simulink model "HydroEye_6DOF_HITL"  (R2024b)
settings: Solver=VariableStepAuto  StartTime=0.0  StopTime=1200  RelTol=1e-3
undefined symbols (not defined in the file): alpha_vec_Cn0, b, b_ref, beta_vec_Cn0, c, CD_flaps, CDo_CD_elev, cg, CL_flaps, Clbeta, Clda, CLo_CL_elev, Clo_Cl_rudder, Clp, Clr, Cm0, Cm_flaps, Cmda, Cmde, Cmo_Cm_elev, Cmq, Cn0, Cnda, Cno_Cn_rudder, Cnp, Cnr, contact, control, cp, CX0, CXda, CXde, CYbeta, CYda, Cyo_Cy_rudder, CZ0, CZda, CZde, d_ref, Earth, F, fractalcoef, Light, m_to_mm, mass, MIL, ms_to_cms, Payload, ref_height, ref_lat, ref_lon, SampleTime, uT_to_gauss, WGS84
libraries: uavmavlinklib x7, simulink_extras x4, aerolibwind2 x3, aerolibatmos2 x2, aerolibasang x2, px4MAVLinkBridgelib x2, shared6dof x1, aerolibadyn x1, simulink x1, aerolibtransform2 x1, sensorgpslib x1, robotcorelib x1
(part 2 of 2)

== system HydroEye_6DOF_HITL/HydroEye Dynamics/Aerodynamics/Aerodynamic Coefficients/Actuator Increments ==
  Alpha : Inport  Unit=deg
  "Actuator Deflections " : Inport  Port=2  Unit=deg
  (0 to inf) Constants Held fixed for alpha<0 : Saturate  UpperLimit=inf  LowerLimit=0
  Ailerons : Subsystem
  AlphaLookup : PreLookup  BreakpointsData=alpha_vec_0  BeginIndexSearchUsingPreviousIndexResult=on  ExtrapMethod=Linear
  AlphaLookup0 : PreLookup  BreakpointsData=alpha_vec_0  BeginIndexSearchUsingPreviousIndexResult=on  ExtrapMethod=Linear
  Bus Creator : BusCreator  Inputs=2
  Bus Creator1 : BusCreator  Inputs=2
  Ruddervators : Subsystem
  Sum : Sum  InputSameDT=on  SaturateOnIntegerOverflow=on  OutDataTypeStr=Inherit: Same as first input
  cl : Outport  InitialOutput=0  VectorParamsAs1DForOutWhenUnconnected=off
  wires:
  Bus Creator/1 -> Ailerons/1(Alpha)
  (0 to inf) Constants Held fixed for alpha<0/1 -> AlphaLookup0/1
  "Actuator Deflections "/1 -> Ailerons/2(Actuators), Ruddervators/2(Actuators)
  Alpha/1 -> (0 to inf) Constants Held fixed for alpha<0/1, AlphaLookup/1
  Ailerons/1(delCoeff) -> Sum/1
  Ruddervators/1(delCoeff) -> Sum/2
  Sum/1 -> cl/1
  Bus Creator1/1 -> Ruddervators/1(Alpha)
  AlphaLookup0/1 -> Bus Creator/1  "k"
  AlphaLookup0/2 -> Bus Creator/2  "f"
  AlphaLookup/1 -> Bus Creator1/1  "k"
  AlphaLookup/2 -> Bus Creator1/2  "f"

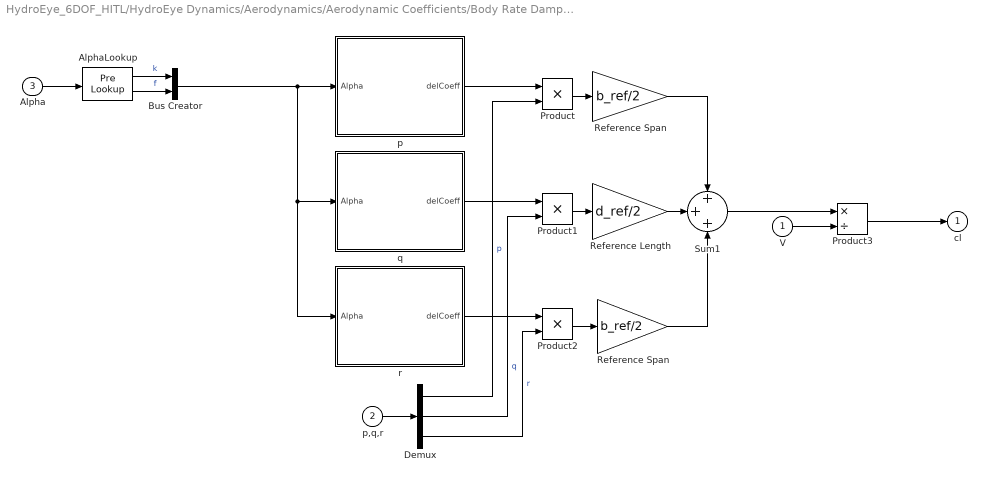
== system HydroEye_6DOF_HITL/HydroEye Dynamics/Aerodynamics/Aerodynamic Coefficients/Body Rate Damping ==
  V : Inport  Unit=m/s
  p,q,r : Inport  Port=2  Unit=rad/second
  Alpha : Inport  Port=3  Unit=deg
  AlphaLookup : PreLookup  BreakpointsData=alpha_vec_damping  BeginIndexSearchUsingPreviousIndexResult=on  ExtrapMethod=Linear
  Bus Creator : BusCreator  Inputs=2
  Demux : Demux  Outputs=3
      settings: DisplayOption=none
  Product : Product  InputSameDT=on  SaturateOnIntegerOverflow=on  OutDataTypeStr=Inherit: Same as first input
  Product1 : Product  InputSameDT=on  SaturateOnIntegerOverflow=on  OutDataTypeStr=Inherit: Same as first input
  Product2 : Product  InputSameDT=on  SaturateOnIntegerOverflow=on  OutDataTypeStr=Inherit: Same as first input
  Product3 : Product  Inputs=*/  InputSameDT=on  SaturateOnIntegerOverflow=on  OutDataTypeStr=Inherit: Same as first input
  Reference Length : Gain  Gain=d_ref/2  SaturateOnIntegerOverflow=on  OutDataTypeStr=Inherit: Same as input  ParamDataTypeStr=Inherit: Same as input
  Reference Span : Gain  Gain=b_ref/2  SaturateOnIntegerOverflow=on  OutDataTypeStr=Inherit: Same as input  ParamDataTypeStr=Inherit: Same as input
  "Reference Span " : Gain  Gain=b_ref/2  SaturateOnIntegerOverflow=on  OutDataTypeStr=Inherit: Same as input  ParamDataTypeStr=Inherit: Same as input
  Sum1 : Sum  Inputs=+++  InputSameDT=on  SaturateOnIntegerOverflow=on  OutDataTypeStr=Inherit: Same as first input
  p : Subsystem
  q : Subsystem
  r : Subsystem
  cl : Outport  InitialOutput=0  VectorParamsAs1DForOutWhenUnconnected=off
  wires:
  Alpha/1 -> AlphaLookup/1
  p/1(delCoeff) -> Product/1
  q/1(delCoeff) -> Product1/1
  p,q,r/1 -> Demux/1
  Demux/1 -> Product/2  "p"
  Demux/2 -> Product1/2  "q"
  Demux/3 -> Product2/2  "r"
  Sum1/1 -> Product3/1
  V/1 -> Product3/2
  Product3/1 -> cl/1
  Product1/1 -> Reference Length/1
  Product2/1 -> "Reference Span "/1
  Product/1 -> Reference Span/1
  r/1(delCoeff) -> Product2/1
  Bus Creator/1 -> r/1(Alpha), q/1(Alpha), p/1(Alpha)
  Reference Length/1 -> Sum1/2
  Reference Span/1 -> Sum1/1
  "Reference Span "/1 -> Sum1/3
  AlphaLookup/1 -> Bus Creator/1  "k"
  AlphaLookup/2 -> Bus Creator/2  "f"

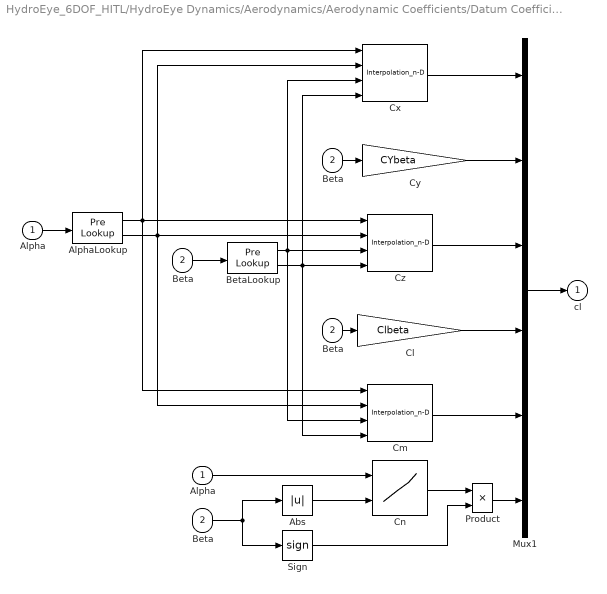
== system HydroEye_6DOF_HITL/HydroEye Dynamics/Aerodynamics/Aerodynamic Coefficients/Datum Coefficients ==
  Alpha : Inport  Unit=deg
  Beta : Inport  Port=2  Unit=deg
  " Cn" : Lookup_n-D  BreakpointsForDimension1=alpha_vec_Cn0  BreakpointsForDimension2=beta_vec_Cn0  Table=Cn0  InternalRulePriority=Speed  RndMeth=Simplest
      settings: InputPortMap=u0,u1
  " Beta" : InportShadow  Port=2  Unit=deg
  " Beta " : InportShadow  Port=2  Unit=deg
  Abs : Abs
  "Alpha " : InportShadow  Unit=deg
  AlphaLookup : PreLookup  BreakpointsData=alpha_vec_0  BeginIndexSearchUsingPreviousIndexResult=on  ExtrapMethod=Linear
  "Beta " : InportShadow  Port=2  Unit=deg
  BetaLookup : PreLookup  BreakpointsData=beta_vec_0  BeginIndexSearchUsingPreviousIndexResult=on  ExtrapMethod=Linear
  Cl : Gain  Gain=Clbeta  SaturateOnIntegerOverflow=on  OutDataTypeStr=Inherit: Same as input  ParamDataTypeStr=Inherit: Same as input
  Cm : Interpolation_n-D  Table=Cm0'  RemoveProtectionIndex=on
  Cx : Interpolation_n-D  Table=CX0'  RemoveProtectionIndex=on
  Cy : Gain  Gain=CYbeta  SaturateOnIntegerOverflow=on  OutDataTypeStr=Inherit: Same as input  ParamDataTypeStr=Inherit: Same as input
  Cz : Interpolation_n-D  Table=CZ0'  RemoveProtectionIndex=on
  Mux1 : Mux  Inputs=6
  Product : Product  InputSameDT=on  SaturateOnIntegerOverflow=on  OutDataTypeStr=Inherit: Same as first input
  Sign : Signum
  cl : Outport  InitialOutput=0  VectorParamsAs1DForOutWhenUnconnected=off
  wires:
  Sign/1 -> Product/2
  " Cn"/1 -> Product/1
  Product/1 -> Mux1/6
  Abs/1 -> " Cn"/2
  Mux1/1 -> cl/1
  Cx/1 -> Mux1/1
  Cz/1 -> Mux1/3
  Cm/1 -> Mux1/5
  Cy/1 -> Mux1/2
  Cl/1 -> Mux1/4
  Alpha/1 -> AlphaLookup/1
  Beta/1 -> BetaLookup/1
  AlphaLookup/1 -> Cz/1, Cm/1, Cx/1
  BetaLookup/1 -> Cz/3, Cx/3, Cm/3
  AlphaLookup/2 -> Cx/2, Cm/2, Cz/2
  "Beta "/1 -> Cy/1
  "Alpha "/1 -> " Cn"/1
  " Beta"/1 -> Abs/1, Sign/1
  " Beta "/1 -> Cl/1
  BetaLookup/2 -> Cz/4, Cx/4, Cm/4

== system HydroEye_6DOF_HITL/HydroEye Dynamics/Ground Model/Crash Detector/norm1 ==
  F : Inport
  Dot Product : DotProduct  OutDataTypeStr=Inherit: Inherit via internal rule
  Sqrt : Sqrt
  Out1 : Outport
  wires:
  Dot Product/1 -> Sqrt/1
  F/1 -> Dot Product/2, Dot Product/1
  Sqrt/1 -> Out1/1

== system HydroEye_6DOF_HITL/HydroEye Dynamics/Ground Model/Friction Force/Soft Coulomb Friction ==
  note: Pennestrì, E., Rossi, V., Salvini, P. et al. Review and comparison of dry friction force models. Nonlinear Dyn 83, 1785–1801 (2016). https://doi.org/10.1007/s11071-015-2485-3
  In1 : Inport
  Tanh : Trigonometry  Operator=tanh
  friction coefficient : Gain  Gain=contact.translation.friction
  vd : Gain  Gain=1/contact.translation.vd
  Out1 : Outport
  wires:
  In1/1 -> vd/1
  vd/1 -> Tanh/1
  Tanh/1 -> friction coefficient/1
  friction coefficient/1 -> Out1/1

== system HydroEye_6DOF_HITL/HydroEye Dynamics/Ground Model/Ground Moment Model/Soft Coulomb Friction ==
  note: Pennestrì, E., Rossi, V., Salvini, P. et al. Review and comparison of dry friction force models. Nonlinear Dyn 83, 1785–1801 (2016). https://doi.org/10.1007/s11071-015-2485-3
  In1 : Inport
  Tanh : Trigonometry  Operator=tanh
  friction coefficient : Gain  Gain=control.rotation.friction
  vd : Gain  Gain=1/control.rotation.vd
  Out1 : Outport
  wires:
  In1/1 -> vd/1
  vd/1 -> Tanh/1
  Tanh/1 -> friction coefficient/1
  friction coefficient/1 -> Out1/1

== system HydroEye_6DOF_HITL/HydroEye Dynamics/Aerodynamics/Aero Coeff/Damping Coeff/p & r ==
  <Angle Rate> : Inport
  <Vb> : Inport  Port=2
  Constant : Constant  Value=[Clp 0 Clr; Cnp 0 Cnr]
  Divide : Product  Inputs=*/
  Dot Product : DotProduct  OutDataTypeStr=Inherit: Inherit via internal rule
  Gain1 : Gain  Gain=b
  Gain2 : Gain  Gain=2
  Matrix Multiply : Product  Multiplication=Matrix(*)
  Radians to Degrees : simulink_extras/Transformations/Radians to Degrees
  Sqrt : Sqrt
  roll rate damping : Outport
  wires:
  Gain2/1 -> Divide/2
  Matrix Multiply/1 -> Gain1/1
  Gain1/1 -> Divide/1
  Divide/1 -> roll rate damping/1  "roll rate damping"
  Constant/1 -> Matrix Multiply/1
  <Vb>/1 -> Dot Product/1, Dot Product/2
  Dot Product/1 -> Sqrt/1
  Sqrt/1 -> Gain2/1
  <Angle Rate>/1 -> Radians to Degrees/1
  Radians to Degrees/1 -> Matrix Multiply/2

== system HydroEye_6DOF_HITL/HydroEye Dynamics/Aerodynamics/Aero Coeff/Damping Coeff/q ==
  <Angle Rate> : Inport
  <Vb> : Inport  Port=2
  Divide : Product  Inputs=*/
  Dot Product : DotProduct  OutDataTypeStr=Inherit: Inherit via internal rule
  Gain : Gain  Gain=Cmq
  Gain1 : Gain  Gain=c
  Gain2 : Gain  Gain=2
  Radians to Degrees : simulink_extras/Transformations/Radians to Degrees
  Selector : Selector  InputPortWidth=3  IndexOptions=Index vector (dialog)  Indices=2  OutputSizes=1
  pitch rate damping : Outport
  wires:
  Selector/1 -> Gain/1
  Gain2/1 -> Divide/2
  Gain/1 -> Gain1/1
  Gain1/1 -> Divide/1
  Divide/1 -> pitch rate damping/1  "pitch rate damping"
  <Vb>/1 -> Dot Product/1, Dot Product/2
  Dot Product/1 -> Gain2/1
  <Angle Rate>/1 -> Radians to Degrees/1
  Radians to Degrees/1 -> Selector/1

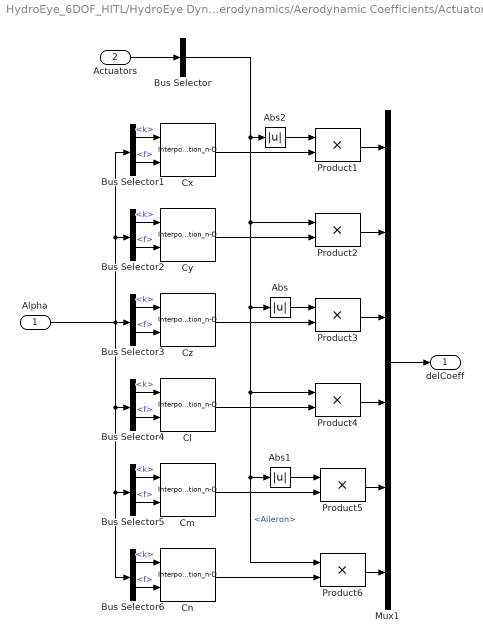
== system HydroEye_6DOF_HITL/HydroEye Dynamics/Aerodynamics/Aerodynamic Coefficients/Actuator Increments/Ailerons ==
  Alpha : Inport
  Actuators : Inport  Port=2
  Abs : Abs
  Abs1 : Abs
  Abs2 : Abs
  Bus Selector : BusSelector  OutputSignals=Aileron
  Bus Selector{1..6} (6 alike) : BusSelector  OutputSignals=k,f
  Cl : Interpolation_n-D  NumberOfTableDimensions=1  Table=Clda  RemoveProtectionIndex=on
      settings: InputPortMap=u0,u1
  Cm : Interpolation_n-D  NumberOfTableDimensions=1  Table=Cmda  RemoveProtectionIndex=on
      settings: InputPortMap=u0,u1
  Cn : Interpolation_n-D  NumberOfTableDimensions=1  Table=Cnda  RemoveProtectionIndex=on
      settings: InputPortMap=u0,u1
  Cx : Interpolation_n-D  NumberOfTableDimensions=1  Table=CXda  RemoveProtectionIndex=on
      settings: InputPortMap=u0,u1
  Cy : Interpolation_n-D  NumberOfTableDimensions=1  Table=CYda  RemoveProtectionIndex=on
      settings: InputPortMap=u0,u1
  Cz : Interpolation_n-D  NumberOfTableDimensions=1  Table=CZda  RemoveProtectionIndex=on
      settings: InputPortMap=u0,u1
  Mux1 : Mux  Inputs=6
  Product{1..6} (6 alike) : Product  InputSameDT=on  SaturateOnIntegerOverflow=on  OutDataTypeStr=Inherit: Same as first input
  delCoeff : Outport  VectorParamsAs1DForOutWhenUnconnected=off
  wires:
  Actuators/1 -> Bus Selector/1
  Mux1/1 -> delCoeff/1
  Product1/1 -> Mux1/1
  Cx/1 -> Product1/2
  Product2/1 -> Mux1/2
  Cy/1 -> Product2/2
  Product3/1 -> Mux1/3
  Cz/1 -> Product3/2
  Cl/1 -> Product4/2
  Product4/1 -> Mux1/4
  Cm/1 -> Product5/2
  Product5/1 -> Mux1/5
  Cn/1 -> Product6/2
  Product6/1 -> Mux1/6
  Bus Selector/1 -> Product6/1, Abs1/1, Product4/1, Abs/1, Product2/1, Abs2/1  "<Aileron>"
  Abs/1 -> Product3/1
  Abs1/1 -> Product5/1
  Abs2/1 -> Product1/1
  Alpha/1 -> Bus Selector1/1, Bus Selector2/1, Bus Selector5/1, Bus Selector6/1, Bus Selector4/1, Bus Selector3/1
  Bus Selector1/1 -> Cx/1  "<k>"
  Bus Selector1/2 -> Cx/2  "<f>"
  Bus Selector2/1 -> Cy/1  "<k>"
  Bus Selector2/2 -> Cy/2  "<f>"
  Bus Selector3/1 -> Cz/1  "<k>"
  Bus Selector3/2 -> Cz/2  "<f>"
  Bus Selector4/1 -> Cl/1  "<k>"
  Bus Selector4/2 -> Cl/2  "<f>"
  Bus Selector5/1 -> Cm/1  "<k>"
  Bus Selector5/2 -> Cm/2  "<f>"
  Bus Selector6/1 -> Cn/1  "<k>"
  Bus Selector6/2 -> Cn/2  "<f>"

== system HydroEye_6DOF_HITL/HydroEye Dynamics/Aerodynamics/Aerodynamic Coefficients/Actuator Increments/Ruddervators ==
  Alpha : Inport
  Actuators : Inport  Port=2
  Bus Selector1 : BusSelector  OutputSignals=Elevator
  Bus Selector2 : BusSelector  OutputSignals=k,f
  Bus Selector3 : BusSelector  OutputSignals=k,f
  Bus Selector5 : BusSelector  OutputSignals=k,f
  Cm : Interpolation_n-D  NumberOfTableDimensions=1  Table=Cmde  RemoveProtectionIndex=on
      settings: InputPortMap=u0,u1
  Constant1 : Constant  Value=0
  Cx : Interpolation_n-D  NumberOfTableDimensions=1  Table=CXde  RemoveProtectionIndex=on
      settings: InputPortMap=u0,u1
  Cz : Interpolation_n-D  NumberOfTableDimensions=1  Table=CZde  RemoveProtectionIndex=on
      settings: InputPortMap=u0,u1
  Mux1 : Mux  Inputs=6
  Product : Product  InputSameDT=on  SaturateOnIntegerOverflow=on  OutDataTypeStr=Inherit: Same as first input
  delCoeff : Outport  VectorParamsAs1DForOutWhenUnconnected=off
  wires:
  Product/1 -> delCoeff/1
  Mux1/1 -> Product/1
  Alpha/1 -> Bus Selector2/1, Bus Selector3/1, Bus Selector5/1
  Cx/1 -> Mux1/1
  Cz/1 -> Mux1/3
  Cm/1 -> Mux1/5
  Constant1/1 -> Mux1/2, Mux1/4, Mux1/6
  Actuators/1 -> Bus Selector1/1
  Bus Selector1/1 -> Product/2  "<Elevator>"
  Bus Selector2/1 -> Cx/1  "<k>"
  Bus Selector2/2 -> Cx/2  "<f>"
  Bus Selector3/1 -> Cz/1  "<k>"
  Bus Selector3/2 -> Cz/2  "<f>"
  Bus Selector5/1 -> Cm/1  "<k>"
  Bus Selector5/2 -> Cm/2  "<f>"

== system HydroEye_6DOF_HITL/HydroEye Dynamics/Aerodynamics/Aerodynamic Coefficients/Body Rate Damping/p ==
  Alpha : Inport
  Bus Selector : BusSelector  OutputSignals=k,f
  Bus Selector1 : BusSelector  OutputSignals=k,f
  Cl : Interpolation_n-D  NumberOfTableDimensions=1  Table=Clp  RemoveProtectionIndex=on
      settings: InputPortMap=u0,u1
  Cn : Interpolation_n-D  NumberOfTableDimensions=1  Table=Cnp  RemoveProtectionIndex=on
      settings: InputPortMap=u0,u1
  Constant1 : Constant  Value=0
  Mux1 : Mux  Inputs=6
  delCoeff : Outport  VectorParamsAs1DForOutWhenUnconnected=off
  wires:
  Mux1/1 -> delCoeff/1
  Constant1/1 -> Mux1/1, Mux1/5, Mux1/3, Mux1/2  "Cxp"
  Cn/1 -> Mux1/6
  Cl/1 -> Mux1/4  "Cl"
  Alpha/1 -> Bus Selector/1, Bus Selector1/1
  Bus Selector/1 -> Cl/1  "<k>"
  Bus Selector/2 -> Cl/2  "<f>"
  Bus Selector1/1 -> Cn/1  "<k>"
  Bus Selector1/2 -> Cn/2  "<f>"

== system HydroEye_6DOF_HITL/HydroEye Dynamics/Aerodynamics/Aerodynamic Coefficients/Body Rate Damping/q ==
  Alpha : Inport
  Bus Selector1 : BusSelector  OutputSignals=k,f
  Cmq : Interpolation_n-D  NumberOfTableDimensions=1  Table=Cmq  RemoveProtectionIndex=on
      settings: InputPortMap=u0,u1
  Constant3 : Constant  Value=0
  Mux1 : Mux  Inputs=6
  delCoeff : Outport  VectorParamsAs1DForOutWhenUnconnected=off
  wires:
  Cmq/1 -> Mux1/5
  Constant3/1 -> Mux1/1, Mux1/2, Mux1/3, Mux1/6, Mux1/4
  Mux1/1 -> delCoeff/1
  Alpha/1 -> Bus Selector1/1
  Bus Selector1/1 -> Cmq/1  "<k>"
  Bus Selector1/2 -> Cmq/2  "<f>"

== system HydroEye_6DOF_HITL/HydroEye Dynamics/Aerodynamics/Aerodynamic Coefficients/Body Rate Damping/r ==
  Alpha : Inport
  Bus Selector : BusSelector  OutputSignals=k,f
  Bus Selector1 : BusSelector  OutputSignals=k,f
  Cl : Interpolation_n-D  NumberOfTableDimensions=1  Table=Clr  RemoveProtectionIndex=on
      settings: InputPortMap=u0,u1
  Cn : Interpolation_n-D  NumberOfTableDimensions=1  Table=Cnr  RemoveProtectionIndex=on
      settings: InputPortMap=u0,u1
  Constant : Constant  Value=0
  Mux1 : Mux  Inputs=6
  delCoeff : Outport  VectorParamsAs1DForOutWhenUnconnected=off
  wires:
  Cn/1 -> Mux1/6
  Cl/1 -> Mux1/4  "Cl"
  Constant/1 -> Mux1/1, Mux1/2, Mux1/5, Mux1/3  "Cxr"
  Mux1/1 -> delCoeff/1
  Alpha/1 -> Bus Selector1/1, Bus Selector/1
  Bus Selector/1 -> Cl/1  "<k>"
  Bus Selector/2 -> Cl/2  "<f>"
  Bus Selector1/1 -> Cn/1  "<k>"
  Bus Selector1/2 -> Cn/2  "<f>"
